simulink library "mfcm_block_lib_v1"  (Simulink 6.1)
undefined symbols (not defined in the file or in its folder): calc_path_data, mfcm_add_phase_noise, mfcm_delay_line_depth, mfcm_dpram_format_init, mfcm_dpram_format_lsb, mfcm_dpram_format_width, mfcm_matrix_rom, mfcm_phase_noise_pacc, mfcm_phase_noise_pinc, mfcm_spectrum_roms
libraries: xbsIndex_r4 x234, mfcm_misc_lib_v1 x8, mfcm_block_lib_v1 x4, mfcm_vector_lib_v1 x3, xbsCopyrightNotice_r4 x1
(part 1 of 3)
settings Model: Creator=dandrews  LastModifiedBy=alexc

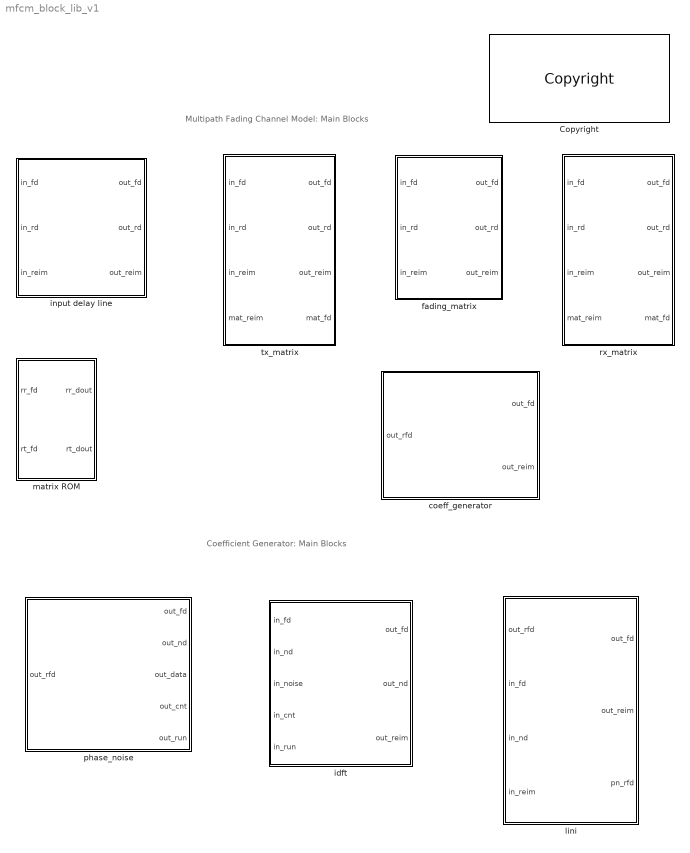
== system mfcm_block_lib_v1 ==
  note: Multipath Fading Channel Model: Main Blocks
  note: Coefficient Generator: Main Blocks
  Copyright : xbsCopyrightNotice_r4/Copyright
  coeff_generator : Subsystem  mask{RATE=32, OUT_WIDTH=18, OUT_BINPT=15, TRIG_WIDTH=18, SPEC_DATA=calc_path_data([2 2 2 2],[1 1 1 1]), SPEC_WIDTH=17, SPEC_BINPT=16, SEED='461AF8228C9F8C92', N_OSC=64, N_IDFT=8192}
      mask prompts: OUT_WIDTH "Output Width"; OUT_BINPT "Output Binary Point"; TRIG_WIDTH "Twiddle Factor Width"; SPEC_DATA "Spectrum Data"; SPEC_WIDTH "Spectrum Width"; SPEC_BINPT "Spectrum Binary Point"; SEED "Random Seed"
      mask Display:
      | disp(sprintf('z^{-14}\nPATHS=%d',prod(size(SPEC_DATA))),'texmode','on');
      | 
      | port_label('input',1,'out_rfd');
      | 
      | port_label('output',1,'out_fd');
      | port_label('output',2,'out_reim');
  fading_matrix : Subsystem  mask{RATE=64, DATAPATH_WIDTH=18, OUT_BINPT=15, SPEC_DATA=calc_path_data([1],[1]), SEED='461AF8228C9F8C92'}
      mask prompts: DATAPATH_WIDTH "Datapath Width"; OUT_BINPT "Output Binary Point"; SPEC_DATA "Spectrum Data"; SEED "Random Seed"
  idft : Subsystem  mask{OUT_WIDTH=18, OUT_BINPT=15, TRIG_WIDTH=18, SPEC_DATA=calc_path_data([3 2 1 0],[1 1 1 1]), SPEC_WIDTH=17, SPEC_BINPT=16, N_OSC=64, N_IDFT=8192}
      mask prompts: OUT_WIDTH "Output Width"; OUT_BINPT "Output Binary Point"; TRIG_WIDTH "Twiddle Factor Width"; SPEC_DATA "Spectrum Data"; SPEC_WIDTH "Spectrum Width"; SPEC_BINPT "Spectrum Binary Point"
  input delay line : Subsystem  mask{MT=4, DELAY=[0 1 2]}
      mask prompts: MT "Number of Transmit Antennas"; DELAY "Path Delay Vector"
  lini : Subsystem  mask{RATE=64, OUT_WIDTH=18, OUT_BINPT=15, CHANNELS=16}
      mask prompts: OUT_WIDTH "Output Width"; OUT_BINPT "Output Binary Point"; CHANNELS "Number Of Channels"
  matrix ROM : Subsystem  mask{MATS=mfcm_matrix_rom(eye(4),1,eye(4)), DATAPATH_WIDTH=18, MAT_BINPT=17}
      mask prompts: MATS "Matrix ROM Data"; DATAPATH_WIDTH "Datapath Width in Bits"; MAT_BINPT "Transmit/Receive Matrix Binary Point"
      mask Display:
      | disp('z^{-3}','texmode','on');
      | 
      | port_label('input',1,'rr_fd');
      | port_label('input',2,'rt_fd');
      | port_label('output',1,'rr_dout');
      | port_label('output',2,'rt_dout');
  phase_noise : Subsystem  mask{SPEC_DATA=calc_path_data([3 2 1 0],[1 1 1 1]), SEED='461AF8228C9F8C92', N_OSC=64, N_IDFT=8192}
      mask prompts: SPEC_DATA "Spectrum Data (with phase noise)"; SEED "Random Seed"
  rx_matrix : Subsystem  mask{MR=4, N=3, BYPASS=0, WIDTH=18, BINPT=15}
      mask prompts: MR "Number of Rx Antennas"; N "Number of Paths"; WIDTH "Output Width"; BINPT "Output Binary Point"
  tx_matrix : Subsystem  mask{MT=4, N=3, BYPASS=0, WIDTH=18, BINPT=17}
      mask prompts: MT "Number of Tx Antennas"; N "Number of Paths"; WIDTH "Output Width"; BINPT "Output Binary Point"

== system mfcm_block_lib_v1/coeff_generator ==
  out_rfd : Inport  Port=1  LatchInput=off
  " Copyright" : Subsystem  mask(Xilinx Digital Up Converter Copyright){}
      mask init:
      | iPos = get_param(gcb,'Position');
      | iWidth=iPos(3)-iPos(1); iHeight=iPos(4)-iPos(2);
      | iCx=iWidth/2;
      | iCy=iHeight/2;
      | [logoX, logoY] = xlogo(iPos);
      mask Display: patch(logoX,logoY, [0.56 0.36 0.27]);
  idft : mfcm_block_lib_v1/idft  OUT_WIDTH=OUT_WIDTH  OUT_BINPT=OUT_BINPT  TRIG_WIDTH=TRIG_WIDTH  SPEC_DATA=SPEC_DATA  SPEC_WIDTH=SPEC_WIDTH  SPEC_BINPT=SPEC_BINPT  N_OSC=N_OSC  N_IDFT=N_IDFT
  lini : mfcm_block_lib_v1/lini  RATE=RATE  OUT_WIDTH=OUT_WIDTH  OUT_BINPT=OUT_BINPT  CHANNELS=prod(size(SPEC_DATA))
  phase_noise : mfcm_block_lib_v1/phase_noise  SPEC_DATA=mfcm_add_phase_noise(SPEC_DATA,SEED)  SEED=SEED  N_OSC=N_OSC  N_IDFT=N_IDFT
  out_fd : Outport
  out_reim : Outport  Port=2
  wires:
  phase_noise/3 -> idft/3
  lini/3 -> phase_noise/1
  out_rfd/1 -> lini/1
  lini/2 -> out_reim/1
  lini/1 -> out_fd/1
  idft/3 -> lini/4
  idft/2 -> lini/3
  idft/1 -> lini/2
  phase_noise/2 -> idft/2
  phase_noise/4 -> idft/4
  phase_noise/1 -> idft/1
  phase_noise/5 -> idft/5

== system mfcm_block_lib_v1/fading_matrix ==
  in_fd : Inport  Port=1  LatchInput=off
  in_rd : Inport  Port=2  LatchInput=off
  in_reim : Inport  Port=3  LatchInput=off
  Terminator : Terminator
  cg : mfcm_block_lib_v1/coeff_generator  RATE=RATE  OUT_WIDTH=DATAPATH_WIDTH  OUT_BINPT=OUT_BINPT  TRIG_WIDTH=DATAPATH_WIDTH  SPEC_DATA=permute(SPEC_DATA,[2 1 3])  SPEC_WIDTH=DATAPATH_WIDTH-1  SPEC_BINPT=DATAPATH_WIDTH-2  SEED=SEED  N_OSC=64  N_IDFT=8192
  fd_pipe : xbsIndex_r4/Delay  en=off  latency=14  dbl_ovrd=off  reg_retiming=off  block_type=delay
      settings: infoedit="Delay line having  configurable length.<P><P>Hardware notes: A delay line is a chain, each link of which is an SRL16 followed by a flip-flop. If register retiming is enabled, the delay line is a chain of flip-flops."  xl_area=[0, 0, 0, 0, 0, 0, 0]  block_version=VER_STRING_GOES_HERE
  multiply SCMAT by SCVEC : mfcm_vector_lib_v1/multiply SCMAT by SCVEC  MAT_H=size(SPEC_DATA,1)*size(SPEC_DATA,3)  MAT_W=size(SPEC_DATA,2)  OUT_WIDTH=DATAPATH_WIDTH  OUT_BINPT=OUT_BINPT
  rd_pipe : xbsIndex_r4/Delay  en=off  latency=14  dbl_ovrd=off  reg_retiming=off  block_type=delay
      settings: infoedit="Delay line having  configurable length.<P><P>Hardware notes: A delay line is a chain, each link of which is an SRL16 followed by a flip-flop. If register retiming is enabled, the delay line is a chain of flip-flops."  xl_area=[0, 0, 0, 0, 0, 0, 0]  block_version=VER_STRING_GOES_HERE
  reim_pipe : xbsIndex_r4/Delay  en=off  latency=14  dbl_ovrd=off  reg_retiming=off  block_type=delay
      settings: infoedit="Delay line having  configurable length.<P><P>Hardware notes: A delay line is a chain, each link of which is an SRL16 followed by a flip-flop. If register retiming is enabled, the delay line is a chain of flip-flops."  xl_area=[0, 0, 0, 0, 0, 0, 0]  block_version=VER_STRING_GOES_HERE
  out_fd : Outport
  out_rd : Outport  Port=2
  out_reim : Outport  Port=3
  wires:
  in_fd/1 -> fd_pipe/1, cg/1
  in_reim/1 -> reim_pipe/1
  in_rd/1 -> rd_pipe/1
  fd_pipe/1 -> multiply SCMAT by SCVEC/1
  rd_pipe/1 -> multiply SCMAT by SCVEC/2
  reim_pipe/1 -> multiply SCMAT by SCVEC/3
  multiply SCMAT by SCVEC/1 -> out_fd/1
  multiply SCMAT by SCVEC/2 -> out_rd/1
  multiply SCMAT by SCVEC/3 -> out_reim/1
  cg/1 -> Terminator/1
  cg/2 -> multiply SCMAT by SCVEC/4

== system mfcm_block_lib_v1/idft ==
  note: iDFT engine has lataency of 8
  in_fd : Inport  Port=1  LatchInput=off
  in_nd : Inport  Port=2  LatchInput=off
  in_noise : Inport  Port=3  LatchInput=off
  in_cnt : Inport  Port=4  LatchInput=off
  in_run : Inport  Port=5  LatchInput=off
  fd_pipe : xbsIndex_r4/Delay  en=off  latency=8+4+2  dbl_ovrd=off  reg_retiming=off  block_type=delay
      settings: infoedit="Delay line having  configurable length.<P><P>Hardware notes: A delay line is a chain, each link of which is an SRL16 followed by a flip-flop. If register retiming is enabled, the delay line is a chain of flip-flops."  xl_area=[0, 0, 0, 0, 0, 0, 0]  block_version=VER_STRING_GOES_HERE
  idft_control : Subsystem
  idft_engine : Subsystem
  nd_pipe : xbsIndex_r4/Delay  en=off  latency=8+4+2  dbl_ovrd=off  reg_retiming=off  block_type=delay
      settings: infoedit="Delay line having  configurable length.<P><P>Hardware notes: A delay line is a chain, each link of which is an SRL16 followed by a flip-flop. If register retiming is enabled, the delay line is a chain of flip-flops."  xl_area=[0, 0, 0, 0, 0, 0, 0]  block_version=VER_STRING_GOES_HERE
  out_pipe : xbsIndex_r4/Delay  en=off  latency=1  dbl_ovrd=off  reg_retiming=off  block_type=delay
      settings: infoedit="Delay line having  configurable length.<P><P>Hardware notes: A delay line is a chain, each link of which is an SRL16 followed by a flip-flop. If register retiming is enabled, the delay line is a chain of flip-flops."  xl_area=[0, 0, 0, 0, 0, 0, 0]  block_version=VER_STRING_GOES_HERE
  safe_mac : mfcm_misc_lib_v1/safe_mac  ACC_GROWTH=log2(N_OSC)  ACC_DEPTH=2
  sat_convert : xbsIndex_r4/Convert  arith_type="Signed  (2's comp)"  n_bits=OUT_WIDTH  bin_pt=OUT_BINPT  quantization=Truncate  overflow=Saturate  latency=1  dbl_ovrd=off  pipeline=off  block_type=convert
      settings: infoedit=The input is presented at the output after quantization and overflow effects.<P><P>Hardware notes: Additional hardware is used when rounding or saturation is selected and output width is less than the input width.  block_version=VER_STRING_GOES_HERE
  out_fd : Outport
  out_nd : Outport  Port=2
  out_reim : Outport  Port=3
  wires:
  idft_engine/4(mac_sub) -> safe_mac/4
  idft_engine/3(mac_acc) -> safe_mac/3
  idft_engine/2(mac_trig) -> safe_mac/2
  idft_engine/1(mac_gain) -> safe_mac/1
  idft_control/3(sin_not_cos) -> idft_engine/3(sin_not_cos)
  idft_control/5(out_kne0) -> idft_engine/5(in_kne0)
  fd_pipe/1 -> out_fd/1
  idft_control/7(out_fd) -> fd_pipe/1
  nd_pipe/1 -> out_nd/1
  idft_control/8(out_kmax) -> nd_pipe/1
  sat_convert/1 -> out_reim/1
  safe_mac/1 -> out_pipe/1
  idft_control/6(out_n) -> idft_engine/6(in_n)
  in_cnt/1 -> idft_control/4(in_cnt)
  in_noise/1 -> idft_control/3(in_noise)
  in_nd/1 -> idft_control/2(in_nd)
  in_fd/1 -> idft_control/1(in_fd)
  idft_control/1(spec_freq) -> idft_engine/1(spec_freq)
  idft_control/4(spec_noise) -> idft_engine/4(spec_noise)
  idft_control/2(spec_path) -> idft_engine/2(spec_path)
  in_run/1 -> idft_control/5(run)
  out_pipe/1 -> sat_convert/1

== system mfcm_block_lib_v1/input delay line ==
  in_fd : Inport  Port=1  LatchInput=off
  in_rd : Inport  Port=2  LatchInput=off
  in_reim : Inport  Port=3  LatchInput=off
  dpram : mfcm_misc_lib_v1/dpram  MEM_DEPTH=mfcm_delay_line_depth(DELAY,MT)  MEM_INIT=0  MEM_MAXDEPTH=16
  pipe0 : xbsIndex_r4/Delay  en=off  latency=2  dbl_ovrd=off  reg_retiming=off  block_type=delay
      settings: infoedit="Delay line having  configurable length.<P><P>Hardware notes: A delay line is a chain, each link of which is an SRL16 followed by a flip-flop. If register retiming is enabled, the delay line is a chain of flip-flops."  xl_area=[0, 0, 0, 0, 0, 0, 0]  block_version=VER_STRING_GOES_HERE
  pipe1 : xbsIndex_r4/Delay  en=on  latency=2  dbl_ovrd=off  reg_retiming=off  block_type=delay
      settings: infoedit="Delay line having  configurable length.<P><P>Hardware notes: A delay line is a chain, each link of which is an SRL16 followed by a flip-flop. If register retiming is enabled, the delay line is a chain of flip-flops."  xl_area=[0, 0, 0, 0, 0, 0, 0]  block_version=VER_STRING_GOES_HERE
  read_control : Subsystem
  write_control : Subsystem
  out_fd : Outport
  out_rd : Outport  Port=2
  out_reim : Outport  Port=3
  wires:
  read_control/3(rd_en) -> pipe1/2
  read_control/2(rd_rd) -> pipe1/1
  pipe1/1 -> out_rd/1
  write_control/1(rd_fd) -> read_control/1(in_fd)
  pipe0/1 -> out_fd/1
  read_control/1(rd_fd) -> pipe0/1
  read_control/4(rd_add) -> dpram/1
  dpram/1 -> out_reim/1
  write_control/4(wr_en) -> dpram/4
  write_control/3(wr_data) -> dpram/3
  write_control/2(wr_add) -> dpram/2
  in_rd/1 -> write_control/2(in_rd)
  in_fd/1 -> write_control/1(in_fd)
  in_reim/1 -> write_control/3(in_reim)

== system mfcm_block_lib_v1/lini ==
  out_rfd : Inport  Port=1  LatchInput=off
  in_fd : Inport  Port=2  LatchInput=off
  in_nd : Inport  Port=3  LatchInput=off
  in_reim : Inport  Port=4  LatchInput=off
  lini_engine : Subsystem
  lini_fifo : Subsystem
  rate_counter : Subsystem
  out_fd : Outport
  out_reim : Outport  Port=2
  pn_rfd : Outport  Port=3
  wires:
  in_fd/1 -> lini_fifo/1(in_fd)
  in_nd/1 -> lini_fifo/2(in_nd)
  in_reim/1 -> lini_fifo/3(in_reim)
  lini_fifo/2(out_re) -> lini_engine/2(in_re)
  lini_fifo/3(out_im) -> lini_engine/3(in_im)
  lini_fifo/5(out_b) -> lini_engine/5(in_b)
  lini_fifo/1(lini_fd) -> lini_engine/1(in_fd)
  lini_engine/1(out_fd) -> out_fd/1
  lini_engine/2(out_reim) -> out_reim/1
  out_rfd/1 -> rate_counter/1(en)
  rate_counter/1(lini_rfd) -> lini_fifo/4(lini_rfd)
  rate_counter/2(pn_rfd) -> lini_fifo/5(pn_rfd), pn_rfd/1
  lini_fifo/6(pn_fd) -> lini_engine/6(pn_fd)
  lini_fifo/4(valid) -> lini_engine/4(in_valid)

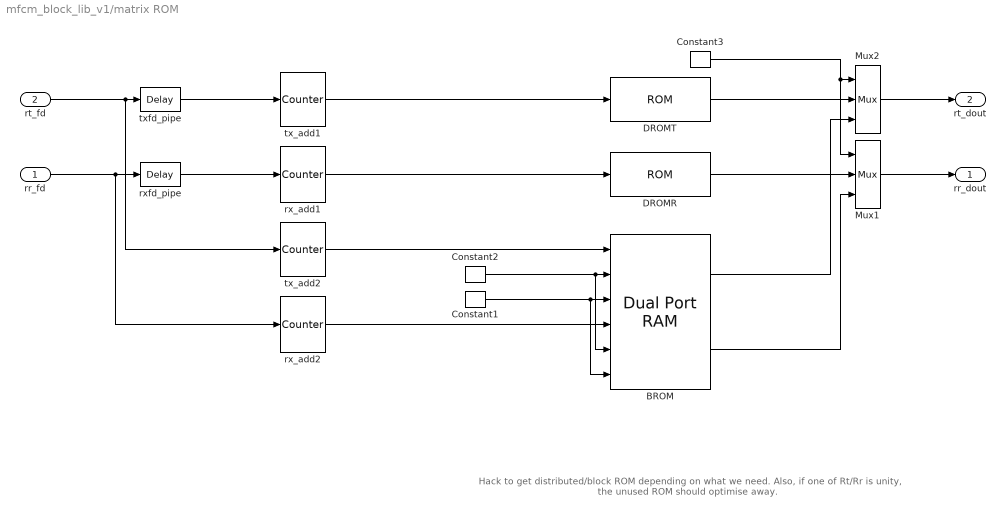
== system mfcm_block_lib_v1/matrix ROM ==
  note: Hack to get distributed/block ROM depending on what we need.
      | Also, if one of Rt/Rr is unity, the unused ROM should optimise away.
  rr_fd : Inport  Port=1  LatchInput=off
  rt_fd : Inport  Port=2  LatchInput=off
  BROM : xbsIndex_r4/Dual Port RAM  depth=2^ceil(log2(max(length(MATS.brom),2)))  initVector=MATS.brom  distributed_mem=Block RAM  init_a=0  init_b=0  rst_a=off  rst_b=off  en_a=off  en_b=off  latency=2  write_mode_A=Read After Write  write_mode_B=Read After Write  dbl_ovrd=off  use_rpm=on  block_type=dpram
      settings: block_version=VER_STRING_GOES_HERE
  Constant1 : xbsIndex_r4/Constant  arith_type=Boolean  const=0  n_bits=1  bin_pt=0  explicit_period=off  period=1  equ=P=C  opselect=C  inp2=PCIN>>17  opr=+  inp1=P  carry=CIN  dbl_ovrd=off  block_type=constant
      settings: block_version=VER_STRING_GOES_HERE
  Constant2 : xbsIndex_r4/Constant  arith_type=Signed (2's comp)  const=0  n_bits=DATAPATH_WIDTH  bin_pt=MAT_BINPT  explicit_period=off  period=1  equ=P=C  opselect=C  inp2=PCIN>>17  opr=+  inp1=P  carry=CIN  dbl_ovrd=off  block_type=constant
      settings: block_version=VER_STRING_GOES_HERE
  Constant3 : xbsIndex_r4/Constant  arith_type=Boolean  const=double(MATS.use_bram~=0)  n_bits=1  bin_pt=0  explicit_period=off  period=1  equ=P=C  opselect=C  inp2=PCIN>>17  opr=+  inp1=P  carry=CIN  dbl_ovrd=off  block_type=constant
      settings: block_version=VER_STRING_GOES_HERE
  DROMR : xbsIndex_r4/ROM  depth=2^ceil(log2(max(length(MATS.dromr),2)))  initVector=MATS.dromr  distributed_mem=Distributed memory  rst=off  init_reg=0  en=off  latency=1  arith_type="Signed  (2's comp)"  n_bits=DATAPATH_WIDTH  bin_pt=MAT_BINPT  dbl_ovrd=off  use_rpm=on  block_type=sprom
      settings: xl_area=[0, 0, 0, 0, 0, 0, 0]  block_version=VER_STRING_GOES_HERE
  DROMT : xbsIndex_r4/ROM  depth=2^ceil(log2(max(length(MATS.dromt),2)))  initVector=MATS.dromt  distributed_mem=Distributed memory  rst=off  init_reg=0  en=off  latency=1  arith_type="Signed  (2's comp)"  n_bits=DATAPATH_WIDTH  bin_pt=MAT_BINPT  dbl_ovrd=off  use_rpm=on  block_type=sprom
      settings: xl_area=[0, 0, 0, 0, 0, 0, 0]  block_version=VER_STRING_GOES_HERE
  Mux1 : xbsIndex_r4/Mux  inputs=2  en=off  latency=0  precision=Full  arith_type=Unsigned  n_bits=8  bin_pt=2  quantization=Truncate  overflow=Wrap  dbl_ovrd=off  block_type=mux
      settings: block_version=VER_STRING_GOES_HERE
  Mux2 : xbsIndex_r4/Mux  inputs=2  en=off  latency=0  precision=Full  arith_type=Unsigned  n_bits=8  bin_pt=2  quantization=Truncate  overflow=Wrap  dbl_ovrd=off  block_type=mux
      settings: block_version=VER_STRING_GOES_HERE
  rx_add1 : xbsIndex_r4/Counter  cnt_type=Free Running  cnt_to=0  operation=Up  start_count=0  cnt_by_val=1  arith_type=Unsigned  n_bits=ceil(log2(max(length(MATS.dromr),2)))  bin_pt=0  load_pin=off  rst=on  en=off  dbl_ovrd=off  explicit_period=off  period=2  block_type=counter
      settings: infoedit="Configurable up, down and up/down counter.<P><P>Hardware notes: Free running counters are the least expensive in hardware.  A count limited counter is implemented by combining a counter with a comparator."  xl_area=[0, 0, 0, 0, 0, 0, 0]  block_version=VER_STRING_GOES_HERE
  rx_add2 : xbsIndex_r4/Counter  cnt_type=Free Running  cnt_to=0  operation=Up  start_count=MATS.brom_rr  cnt_by_val=1  arith_type=Unsigned  n_bits=ceil(log2(max(length(MATS.brom),2)))  bin_pt=0  load_pin=off  rst=on  en=off  dbl_ovrd=off  explicit_period=off  period=2  block_type=counter
      settings: infoedit="Configurable up, down and up/down counter.<P><P>Hardware notes: Free running counters are the least expensive in hardware.  A count limited counter is implemented by combining a counter with a comparator."  xl_area=[0, 0, 0, 0, 0, 0, 0]  block_version=VER_STRING_GOES_HERE
  rxfd_pipe : xbsIndex_r4/Delay  en=off  latency=1  dbl_ovrd=off  reg_retiming=off  block_type=delay
      settings: infoedit="Delay line having  configurable length.<P><P>Hardware notes: A delay line is a chain, each link of which is an SRL16 followed by a flip-flop. If register retiming is enabled, the delay line is a chain of flip-flops."  block_version=VER_STRING_GOES_HERE
  tx_add1 : xbsIndex_r4/Counter  cnt_type=Free Running  cnt_to=Inf  operation=Up  start_count=0  cnt_by_val=1  arith_type=Unsigned  n_bits=ceil(log2(max(length(MATS.dromt),2)))  bin_pt=0  load_pin=off  rst=on  en=off  dbl_ovrd=off  explicit_period=off  period=2  block_type=counter
      settings: infoedit="Configurable up, down and up/down counter.<P><P>Hardware notes: Free running counters are the least expensive in hardware.  A count limited counter is implemented by combining a counter with a comparator."  xl_area=[0, 0, 0, 0, 0, 0, 0]  block_version=VER_STRING_GOES_HERE
  tx_add2 : xbsIndex_r4/Counter  cnt_type=Free Running  cnt_to=Inf  operation=Up  start_count=MATS.brom_rt  cnt_by_val=1  arith_type=Unsigned  n_bits=ceil(log2(max(length(MATS.brom),2)))  bin_pt=0  load_pin=off  rst=on  en=off  dbl_ovrd=off  explicit_period=off  period=2  block_type=counter
      settings: infoedit="Configurable up, down and up/down counter.<P><P>Hardware notes: Free running counters are the least expensive in hardware.  A count limited counter is implemented by combining a counter with a comparator."  xl_area=[0, 0, 0, 0, 0, 0, 0]  block_version=VER_STRING_GOES_HERE
  txfd_pipe : xbsIndex_r4/Delay  en=off  latency=1  dbl_ovrd=off  reg_retiming=off  block_type=delay
      settings: infoedit="Delay line having  configurable length.<P><P>Hardware notes: A delay line is a chain, each link of which is an SRL16 followed by a flip-flop. If register retiming is enabled, the delay line is a chain of flip-flops."  block_version=VER_STRING_GOES_HERE
  rr_dout : Outport
  rt_dout : Outport  Port=2
  wires:
  Constant1/1 -> BROM/6, BROM/3
  Constant2/1 -> BROM/5, BROM/2
  DROMR/1 -> Mux1/2
  DROMT/1 -> Mux2/2
  rr_fd/1 -> rx_add2/1, rxfd_pipe/1
  rt_fd/1 -> tx_add2/1, txfd_pipe/1
  rxfd_pipe/1 -> rx_add1/1
  tx_add1/1 -> DROMT/1
  txfd_pipe/1 -> tx_add1/1
  BROM/1 -> Mux2/3
  BROM/2 -> Mux1/3
  Mux2/1 -> rt_dout/1
  Mux1/1 -> rr_dout/1
  rx_add1/1 -> DROMR/1
  Constant3/1 -> Mux2/1, Mux1/1
  tx_add2/1 -> BROM/1
  rx_add2/1 -> BROM/4

== system mfcm_block_lib_v1/phase_noise ==
  note: lfsr must be clocked once per path.
      | Note that this does not need to be synchronised to pn_engine block
      | - if they are not synced there is a very small chance that two increments
      | can be updated per path - this is harmless and on average will be fine.
  out_rfd : Inport  Port=1  LatchInput=off
  Constant1 : xbsIndex_r4/Constant  arith_type=Unsigned  const=1  n_bits=1  bin_pt=0  explicit_period=off  period=1  equ=P=C  opselect=C  inp2=PCIN>>17  opr=+  inp1=P  carry=CIN  dbl_ovrd=off  block_type=constant
      settings: block_version=VER_STRING_GOES_HERE
  Slice : xbsIndex_r4/Slice  nbits=ceil(log2(2*N_OSC))  boolean_output=off  mode=Lower Bit Location + Width  bit1=0  base1=MSB of Input  bit0=0  base0=LSB of Input  dbl_ovrd=off  block_type=slice
      settings: infoedit="Extracts a given range of bits from each input sample and presents it at the output.  The output type is ordinarily unsigned with binary point at zero, but can be Boolean when the slice is one bit wide.<P><P>Hardware notes: In hardware this block costs nothing."  block_version=VER_STRING_GOES_HERE
  lfsr1 : Subsystem  mask{SEED=SEED}
      mask prompts: SEED "Seed value (16 hex digits)"
  lfsr_relop : xbsIndex_r4/Relational  mode=a=b  en=off  latency=1  dbl_ovrd=off  block_type=relational
      settings: xl_area=[0, 0, 0, 0, 0, 0, 0]  block_version=VER_STRING_GOES_HERE
  pn_engine : Subsystem
  out_fd : Outport
  out_nd : Outport  Port=2
  out_data : Outport  Port=3
  out_cnt : Outport  Port=4
  out_run : Outport  Port=5
  wires:
  pn_engine/5(out_run) -> out_run/1
  pn_engine/1(out_fd) -> out_fd/1
  pn_engine/3(out_data) -> out_data/1
  lfsr1/1(out_data) -> pn_engine/2(noise)
  out_rfd/1 -> pn_engine/1(rfd)
  pn_engine/2(out_nd) -> out_nd/1
  pn_engine/4(out_cnt) -> out_cnt/1, Slice/1
  lfsr_relop/1 -> lfsr1/1(en)
  Constant1/1 -> lfsr_relop/2
  Slice/1 -> lfsr_relop/1

== system mfcm_block_lib_v1/rx_matrix ==
  note: Matrix ROM
      | latency is 3
  note: Bypass path - if RR is unity we don't need all this.
      | Should optimise away
  in_fd : Inport  Port=1  LatchInput=off
  in_rd : Inport  Port=2  LatchInput=off
  in_reim : Inport  Port=3  LatchInput=off
  mat_reim : Inport  Port=4  LatchInput=off
  Constant1 : xbsIndex_r4/Constant  arith_type=Boolean  const=double(BYPASS~=0)  n_bits=1  bin_pt=0  explicit_period=off  period=1  equ=P=C  opselect=C  inp2=PCIN>>17  opr=+  inp1=P  carry=CIN  dbl_ovrd=off  block_type=constant
      settings: block_version=VER_STRING_GOES_HERE
  Convert : xbsIndex_r4/Convert  arith_type="Signed  (2's comp)"  n_bits=WIDTH  bin_pt=BINPT  quantization=Truncate  overflow=Wrap  latency=0  dbl_ovrd=off  pipeline=off  block_type=convert
      settings: infoedit=The input is presented at the output after quantization and overflow effects.<P><P>Hardware notes: Additional hardware is used when rounding or saturation is selected and output width is less than the input width.  xl_area=[0, 0, 0, 0, 0, 0, 0]  block_version=VER_STRING_GOES_HERE
  Mux1 : xbsIndex_r4/Mux  inputs=2  en=off  latency=0  precision=Full  arith_type=Unsigned  n_bits=8  bin_pt=2  quantization=Truncate  overflow=Wrap  dbl_ovrd=off  block_type=mux
      settings: block_version=VER_STRING_GOES_HERE
  Mux2 : xbsIndex_r4/Mux  inputs=2  en=off  latency=0  precision=Full  arith_type=Unsigned  n_bits=8  bin_pt=2  quantization=Truncate  overflow=Wrap  dbl_ovrd=off  block_type=mux
      settings: block_version=VER_STRING_GOES_HERE
  Mux3 : xbsIndex_r4/Mux  inputs=2  en=off  latency=0  precision=Full  arith_type=Unsigned  n_bits=8  bin_pt=2  quantization=Truncate  overflow=Wrap  dbl_ovrd=off  block_type=mux
      settings: block_version=VER_STRING_GOES_HERE
  fd_pipe : xbsIndex_r4/Delay  en=off  latency=3  dbl_ovrd=off  reg_retiming=off  block_type=delay
      settings: infoedit="Delay line having  configurable length.<P><P>Hardware notes: A delay line is a chain, each link of which is an SRL16 followed by a flip-flop. If register retiming is enabled, the delay line is a chain of flip-flops."  xl_area=[0, 0, 0, 0, 0, 0, 0]  block_version=VER_STRING_GOES_HERE
  multiply SCMAT by SCVEC : mfcm_vector_lib_v1/multiply SCMAT by SCVEC  MAT_H=MR  MAT_W=MR*N  OUT_WIDTH=WIDTH  OUT_BINPT=BINPT
  rd_pipe : xbsIndex_r4/Delay  en=off  latency=3  dbl_ovrd=off  reg_retiming=off  block_type=delay
      settings: infoedit="Delay line having  configurable length.<P><P>Hardware notes: A delay line is a chain, each link of which is an SRL16 followed by a flip-flop. If register retiming is enabled, the delay line is a chain of flip-flops."  xl_area=[0, 0, 0, 0, 0, 0, 0]  block_version=VER_STRING_GOES_HERE
  reim_pipe : xbsIndex_r4/Delay  en=off  latency=3  dbl_ovrd=off  reg_retiming=off  block_type=delay
      settings: infoedit="Delay line having  configurable length.<P><P>Hardware notes: A delay line is a chain, each link of which is an SRL16 followed by a flip-flop. If register retiming is enabled, the delay line is a chain of flip-flops."  xl_area=[0, 0, 0, 0, 0, 0, 0]  block_version=VER_STRING_GOES_HERE
  out_fd : Outport
  out_rd : Outport  Port=2
  out_reim : Outport  Port=3
  mat_fd : Outport  Port=4
  wires:
  reim_pipe/1 -> multiply SCMAT by SCVEC/3
  rd_pipe/1 -> multiply SCMAT by SCVEC/2
  in_rd/1 -> rd_pipe/1, Mux1/3
  mat_reim/1 -> multiply SCMAT by SCVEC/4
  in_fd/1 -> fd_pipe/1, Mux2/3, mat_fd/1
  in_reim/1 -> reim_pipe/1, Convert/1
  fd_pipe/1 -> multiply SCMAT by SCVEC/1
  multiply SCMAT by SCVEC/1 -> Mux2/2
  multiply SCMAT by SCVEC/2 -> Mux1/2
  multiply SCMAT by SCVEC/3 -> Mux3/2
  Constant1/1 -> Mux1/1, Mux3/1, Mux2/1
  Mux2/1 -> out_fd/1
  Mux1/1 -> out_rd/1
  Mux3/1 -> out_reim/1
  Convert/1 -> Mux3/3

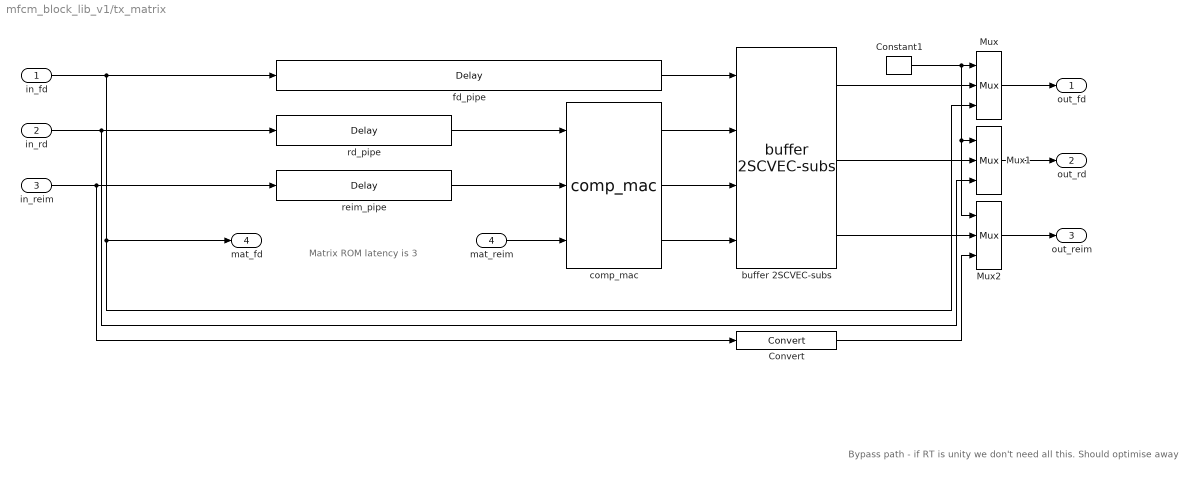
== system mfcm_block_lib_v1/tx_matrix ==
  note: Matrix ROM
      | latency is 3
  note: Bypass path - if RT is unity we don't need all this.
      | Should optimise away
  in_fd : Inport  Port=1  LatchInput=off
  in_rd : Inport  Port=2  LatchInput=off
  in_reim : Inport  Port=3  LatchInput=off
  mat_reim : Inport  Port=4  LatchInput=off
  Constant1 : xbsIndex_r4/Constant  arith_type=Boolean  const=double(BYPASS~=0)  n_bits=1  bin_pt=0  explicit_period=off  period=1  equ=P=C  opselect=C  inp2=PCIN>>17  opr=+  inp1=P  carry=CIN  dbl_ovrd=off  block_type=constant
      settings: block_version=VER_STRING_GOES_HERE
  Convert : xbsIndex_r4/Convert  arith_type="Signed  (2's comp)"  n_bits=WIDTH  bin_pt=BINPT  quantization=Truncate  overflow=Wrap  latency=0  dbl_ovrd=off  pipeline=off  block_type=convert
      settings: infoedit=The input is presented at the output after quantization and overflow effects.<P><P>Hardware notes: Additional hardware is used when rounding or saturation is selected and output width is less than the input width.  xl_area=[0, 0, 0, 0, 0, 0, 0]  block_version=VER_STRING_GOES_HERE
  Mux : xbsIndex_r4/Mux  inputs=2  en=off  latency=0  precision=Full  arith_type=Unsigned  n_bits=8  bin_pt=2  quantization=Truncate  overflow=Wrap  dbl_ovrd=off  block_type=mux
      settings: block_version=VER_STRING_GOES_HERE
  Mux1 : xbsIndex_r4/Mux  inputs=2  en=off  latency=0  precision=Full  arith_type=Unsigned  n_bits=8  bin_pt=2  quantization=Truncate  overflow=Wrap  dbl_ovrd=off  block_type=mux
      settings: block_version=VER_STRING_GOES_HERE
  Mux2 : xbsIndex_r4/Mux  inputs=2  en=off  latency=0  precision=Full  arith_type=Unsigned  n_bits=8  bin_pt=2  quantization=Truncate  overflow=Wrap  dbl_ovrd=off  block_type=mux
      settings: block_version=VER_STRING_GOES_HERE
  buffer 2SCVEC-subs : mfcm_vector_lib_v1/buffer 2SCVEC-subs  SUB_SIZE=MT  SUB_COUNT=N  REP_COUNT=MT
  comp_mac : mfcm_misc_lib_v1/comp_mac  MULS=MT  OUT_WIDTH=WIDTH  OUT_BINPT=BINPT
  fd_pipe : xbsIndex_r4/Delay  en=off  latency=3+2*MT+8  dbl_ovrd=off  reg_retiming=off  block_type=delay
      settings: infoedit="Delay line having  configurable length.<P><P>Hardware notes: A delay line is a chain, each link of which is an SRL16 followed by a flip-flop. If register retiming is enabled, the delay line is a chain of flip-flops."  xl_area=[0, 0, 0, 0, 0, 0, 0]  block_version=VER_STRING_GOES_HERE
  rd_pipe : xbsIndex_r4/Delay  en=off  latency=3  dbl_ovrd=off  reg_retiming=off  block_type=delay
      settings: infoedit="Delay line having  configurable length.<P><P>Hardware notes: A delay line is a chain, each link of which is an SRL16 followed by a flip-flop. If register retiming is enabled, the delay line is a chain of flip-flops."  xl_area=[0, 0, 0, 0, 0, 0, 0]  block_version=VER_STRING_GOES_HERE
  reim_pipe : xbsIndex_r4/Delay  en=off  latency=3  dbl_ovrd=off  reg_retiming=off  block_type=delay
      settings: infoedit="Delay line having  configurable length.<P><P>Hardware notes: A delay line is a chain, each link of which is an SRL16 followed by a flip-flop. If register retiming is enabled, the delay line is a chain of flip-flops."  xl_area=[0, 0, 0, 0, 0, 0, 0]  block_version=VER_STRING_GOES_HERE
  out_fd : Outport
  out_rd : Outport  Port=2
  out_reim : Outport  Port=3
  mat_fd : Outport  Port=4
  wires:
  in_reim/1 -> reim_pipe/1, Convert/1
  buffer 2SCVEC-subs/1 -> Mux/2
  buffer 2SCVEC-subs/2 -> Mux1/2
  buffer 2SCVEC-subs/3 -> Mux2/2
  in_fd/1 -> fd_pipe/1, Mux/3, mat_fd/1
  mat_reim/1 -> comp_mac/3
  in_rd/1 -> rd_pipe/1, Mux1/3
  rd_pipe/1 -> comp_mac/1
  reim_pipe/1 -> comp_mac/2
  fd_pipe/1 -> buffer 2SCVEC-subs/1
  comp_mac/1 -> buffer 2SCVEC-subs/2
  comp_mac/2 -> buffer 2SCVEC-subs/3
  comp_mac/3 -> buffer 2SCVEC-subs/4
  Constant1/1 -> Mux1/1, Mux2/1, Mux/1
  Mux/1 -> out_fd/1
  Mux1/1 -> out_rd/1
  Mux2/1 -> out_reim/1
  Convert/1 -> Mux2/3

== system mfcm_block_lib_v1/coeff_generator/ Copyright ==
  note: -- Copyright(C) 2005 by Xilinx, Inc. All rights reserved.
      |  -- This text/file contains proprietary, confidential
      |  -- information of Xilinx, Inc., is distributed under license
      |  -- from Xilinx, Inc., and may be used, copied and/or
      |  -- disclosed only pursuant to the terms of a valid license
      |  -- agreement with Xilinx, Inc. Xilinx hereby grants you
      |  -- a license to use this text/file solely for design, simulation,
      |  -- implementation and creation of design files limited
      |  -- to Xilinx devices or technologies. Use with non-Xilinx
      |  -- devices or technologies is expressly prohibited and
      |  -- immediately terminates your license unless covered by
      |  -- a separate agreement.
      |  --
      |  -- Xilinx is providing this design, code, or information
      |  -- "as is" solely for use in developing programs and
      |  -- solutions for Xilinx devices. By providing this design,
      |  -- code, or information as one possible implementation of
      |  -- this feature, application or standard, Xilinx is making no
      |  -- representation that this implementation is free from any
      |  -- claims of infringement. You are responsible for
      |  -- obtaining any rights you may require for your implementation.
      |  -- Xilinx expressly disclaims any warranty whatsoever with
      |  -- respect to the adequacy of the implementation, including
      |  -- but not limited to any warranties or representations that this
      |  -- implementation is free from claims of infringement, implied
      |  -- warranties of merchantability or fitness for a particular
      |  -- purpose.
      |  --
      |  -- Xilinx products are not intended for use in life support
      |  -- appliances, devices, or systems. Use in such applications are
      |  -- expressly prohibited.
      |  --
      |  -- This copyright and support notice must be retained as part
      |  -- of this text at all times. (c) Copyright 1995-2005 Xilinx, Inc.
      |  -- All rights reserved.

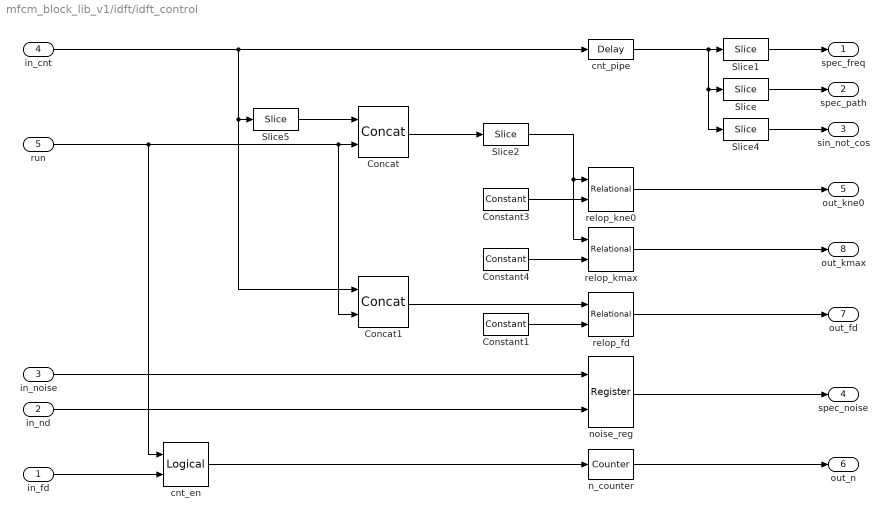
== system mfcm_block_lib_v1/idft/idft_control ==
  in_fd : Inport  Port=1  LatchInput=off
  in_nd : Inport  Port=2  LatchInput=off
  in_noise : Inport  Port=3  LatchInput=off
  in_cnt : Inport  Port=4  LatchInput=off
  run : Inport  Port=5  LatchInput=off
  Concat : xbsIndex_r4/Concat  num_inputs=2  dbl_ovrd=off  block_type=concat
      settings: block_version=VER_STRING_GOES_HERE
  Concat1 : xbsIndex_r4/Concat  num_inputs=2  dbl_ovrd=off  block_type=concat
      settings: block_version=VER_STRING_GOES_HERE
  Constant1 : xbsIndex_r4/Constant  arith_type=Unsigned  const=2*(2^ceil(log2(2*N_OSC*prod(size(SPEC_DATA))))-2*N_OSC*prod(size(SPEC_DATA))+2*N_OSC-2)+1  n_bits=ceil(log2(2*N_OSC*prod(size(SPEC_DATA))))+1  bin_pt=0  explicit_period=off  period=1  equ=P=C  opselect=C  inp2=PCIN>>17  opr=+  inp1=P  carry=CIN  dbl_ovrd=off  block_type=constant
      settings: block_version=VER_STRING_GOES_HERE
  Constant3 : xbsIndex_r4/Constant  arith_type=Unsigned  const=0+1  n_bits=log2(N_OSC)+1  bin_pt=0  explicit_period=off  period=1  equ=P=C  opselect=C  inp2=PCIN>>17  opr=+  inp1=P  carry=CIN  dbl_ovrd=off  block_type=constant
      settings: block_version=VER_STRING_GOES_HERE
  Constant4 : xbsIndex_r4/Constant  arith_type=Unsigned  const=2*(N_OSC-1)+1  n_bits=log2(N_OSC)+1  bin_pt=0  explicit_period=off  period=1  equ=P=C  opselect=C  inp2=PCIN>>17  opr=+  inp1=P  carry=CIN  dbl_ovrd=off  block_type=constant
      settings: block_version=VER_STRING_GOES_HERE
  Slice : xbsIndex_r4/Slice  nbits=ceil(log2(max(prod(size(SPEC_DATA)),2)))  boolean_output=off  mode=Upper Bit Location + Width  bit1=0  base1=MSB of Input  bit0=0  base0=LSB of Input  dbl_ovrd=off  block_type=slice
      settings: infoedit="Extracts a given range of bits from each input sample and presents it at the output.  The output type is ordinarily unsigned with binary point at zero, but can be Boolean when the slice is one bit wide.<P><P>Hardware notes: In hardware this block costs nothing."  block_version=VER_STRING_GOES_HERE
  Slice1 : xbsIndex_r4/Slice  nbits=log2(N_OSC)  boolean_output=off  mode=Lower Bit Location + Width  bit1=0  base1=MSB of Input  bit0=1  base0=LSB of Input  dbl_ovrd=off  block_type=slice
      settings: infoedit="Extracts a given range of bits from each input sample and presents it at the output.  The output type is ordinarily unsigned with binary point at zero, but can be Boolean when the slice is one bit wide.<P><P>Hardware notes: In hardware this block costs nothing."  block_version=VER_STRING_GOES_HERE
  Slice2 : xbsIndex_r4/Slice  nbits=log2(N_OSC)+1  boolean_output=off  mode=Lower Bit Location + Width  bit1=0  base1=MSB of Input  bit0=0  base0=LSB of Input  dbl_ovrd=off  block_type=slice
      settings: infoedit="Extracts a given range of bits from each input sample and presents it at the output.  The output type is ordinarily unsigned with binary point at zero, but can be Boolean when the slice is one bit wide.<P><P>Hardware notes: In hardware this block costs nothing."  block_version=VER_STRING_GOES_HERE
  Slice4 : xbsIndex_r4/Slice  nbits=1  boolean_output=on  mode=Lower Bit Location + Width  bit1=0  base1=MSB of Input  bit0=0  base0=LSB of Input  dbl_ovrd=off  block_type=slice
      settings: infoedit="Extracts a given range of bits from each input sample and presents it at the output.  The output type is ordinarily unsigned with binary point at zero, but can be Boolean when the slice is one bit wide.<P><P>Hardware notes: In hardware this block costs nothing."  block_version=VER_STRING_GOES_HERE
  Slice5 : xbsIndex_r4/Slice  nbits=ceil(log2(prod(size(SPEC_DATA))*N_OSC))  boolean_output=off  mode=Upper Bit Location + Width  bit1=0  base1=MSB of Input  bit0=1  base0=LSB of Input  dbl_ovrd=off  block_type=slice
      settings: infoedit="Extracts a given range of bits from each input sample and presents it at the output.  The output type is ordinarily unsigned with binary point at zero, but can be Boolean when the slice is one bit wide.<P><P>Hardware notes: In hardware this block costs nothing."  block_version=VER_STRING_GOES_HERE
  cnt_en : xbsIndex_r4/Logical  logical_function=AND  inputs=2  en=off  latency=0  precision=Full  arith_type=Unsigned  n_bits=1  bin_pt=0  align_bp=on  dbl_ovrd=off  block_type=logical
      settings: xl_area=[0, 0, 0, 0, 0, 0, 0]  block_version=VER_STRING_GOES_HERE
  cnt_pipe : xbsIndex_r4/Delay  en=off  latency=1  dbl_ovrd=off  reg_retiming=off  block_type=delay
      settings: infoedit="Delay line having  configurable length.<P><P>Hardware notes: A delay line is a chain, each link of which is an SRL16 followed by a flip-flop. If register retiming is enabled, the delay line is a chain of flip-flops."  xl_area=[0, 0, 0, 0, 0, 0, 0]  block_version=VER_STRING_GOES_HERE
  n_counter : xbsIndex_r4/Counter  cnt_type=Free Running  cnt_to=Inf  operation=Up  start_count=0  cnt_by_val=1  arith_type=Unsigned  n_bits=log2(N_IDFT)  bin_pt=0  load_pin=off  rst=off  en=on  dbl_ovrd=off  explicit_period=off  period=1  block_type=counter
      settings: infoedit="Configurable up, down and up/down counter.<P><P>Hardware notes: Free running counters are the least expensive in hardware.  A count limited counter is implemented by combining a counter with a comparator."  block_version=VER_STRING_GOES_HERE
  noise_reg : xbsIndex_r4/Register  init=0  rst=off  en=on  dbl_ovrd=off  block_type=register
      settings: xl_area=[0, 0, 0, 0, 0, 0, 0]  block_version=VER_STRING_GOES_HERE
  relop_fd : xbsIndex_r4/Relational  mode=a=b  en=off  latency=1  dbl_ovrd=off  block_type=relational
      settings: xl_area=[0, 0, 0, 0, 0, 0, 0]  block_version=VER_STRING_GOES_HERE
  relop_kmax : xbsIndex_r4/Relational  mode=a=b  en=off  latency=1  dbl_ovrd=off  block_type=relational
      settings: xl_area=[0, 0, 0, 0, 0, 0, 0]  block_version=VER_STRING_GOES_HERE
  relop_kne0 : xbsIndex_r4/Relational  mode=a!=b  en=off  latency=1  dbl_ovrd=off  block_type=relational
      settings: xl_area=[0, 0, 0, 0, 0, 0, 0]  block_version=VER_STRING_GOES_HERE
  spec_freq : Outport
  spec_path : Outport  Port=2
  sin_not_cos : Outport  Port=3
  spec_noise : Outport  Port=4
  out_kne0 : Outport  Port=5
  out_n : Outport  Port=6
  out_fd : Outport  Port=7
  out_kmax : Outport  Port=8
  wires:
  n_counter/1 -> out_n/1
  in_fd/1 -> cnt_en/2
  cnt_en/1 -> n_counter/1
  Slice4/1 -> sin_not_cos/1
  Concat1/1 -> relop_fd/1
  Slice5/1 -> Concat/1
  Concat/1 -> Slice2/1
  cnt_pipe/1 -> Slice4/1, Slice/1, Slice1/1
  relop_fd/1 -> out_fd/1
  Constant1/1 -> relop_fd/2
  relop_kmax/1 -> out_kmax/1
  Constant4/1 -> relop_kmax/2
  relop_kne0/1 -> out_kne0/1
  Slice2/1 -> relop_kmax/1, relop_kne0/1
  Constant3/1 -> relop_kne0/2
  in_nd/1 -> noise_reg/2
  noise_reg/1 -> spec_noise/1
  in_noise/1 -> noise_reg/1
  Slice/1 -> spec_path/1
  Slice1/1 -> spec_freq/1
  in_cnt/1 -> Concat1/1, Slice5/1, cnt_pipe/1
  run/1 -> cnt_en/1, Concat1/2, Concat/2

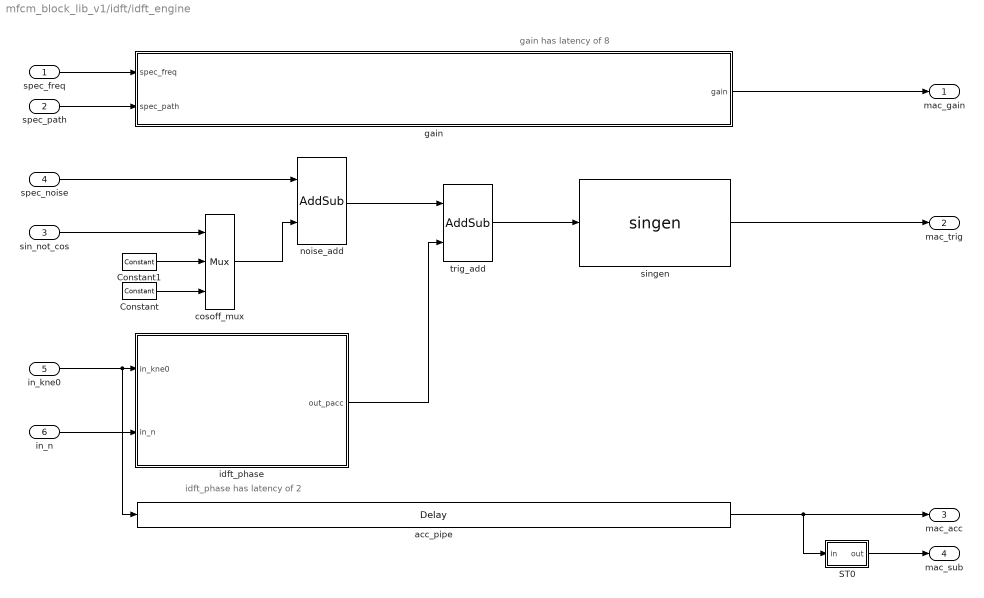
== system mfcm_block_lib_v1/idft/idft_engine ==
  note: idft_phase has latency of 2
  note: gain has latency of 8
  spec_freq : Inport  Port=1  LatchInput=off
  spec_path : Inport  Port=2  LatchInput=off
  sin_not_cos : Inport  Port=3  LatchInput=off
  spec_noise : Inport  Port=4  LatchInput=off
  in_kne0 : Inport  Port=5  LatchInput=off
  in_n : Inport  Port=6  LatchInput=off
  Constant : xbsIndex_r4/Constant  arith_type=Unsigned  const=0  n_bits=log2(N_IDFT)  bin_pt=0  explicit_period=off  period=1  equ=P=C  opselect=C  inp2=PCIN>>17  opr=+  inp1=P  carry=CIN  dbl_ovrd=off  block_type=constant
      settings: block_version=VER_STRING_GOES_HERE
  Constant1 : xbsIndex_r4/Constant  arith_type=Unsigned  const=N_IDFT/4  n_bits=log2(N_IDFT)  bin_pt=0  explicit_period=off  period=1  equ=P=C  opselect=C  inp2=PCIN>>17  opr=+  inp1=P  carry=CIN  dbl_ovrd=off  block_type=constant
      settings: block_version=VER_STRING_GOES_HERE
  ST0 : Subsystem
  acc_pipe : xbsIndex_r4/Delay  en=off  latency=2+1+5  dbl_ovrd=off  reg_retiming=off  block_type=delay
      settings: infoedit="Delay line having  configurable length.<P><P>Hardware notes: A delay line is a chain, each link of which is an SRL16 followed by a flip-flop. If register retiming is enabled, the delay line is a chain of flip-flops."  xl_area=[0, 0, 0, 0, 0, 0, 0]  block_version=VER_STRING_GOES_HERE
  "cosoff_mux " : xbsIndex_r4/Mux  inputs=2  en=off  latency=0  precision=Full  arith_type=Unsigned  n_bits=8  bin_pt=2  quantization=Truncate  overflow=Wrap  dbl_ovrd=off  block_type=mux
      settings: block_version=VER_STRING_GOES_HERE
  gain : Subsystem  mask{ROMS=mfcm_spectrum_roms(SPEC_DATA,N_IDFT)}
      mask prompts: ROMS "Spectrum ROMS"
  idft_phase : Subsystem
  noise_add : xbsIndex_r4/AddSub  mode=Addition  use_carryin=off  use_carryout=off  en=off  latency=2  precision=User Defined  arith_type=Unsigned  n_bits=log2(N_IDFT)  bin_pt=0  quantization=Truncate  overflow=Wrap  dbl_ovrd=off  use_behavioral_HDL=on  pipelined=on  use_rpm=on  block_type=addsub
      settings: xl_area=[0, 0, 0, 0, 0, 0, 0]  block_version=VER_STRING_GOES_HERE
  singen : mfcm_misc_lib_v1/singen  N=N_IDFT  OUT_WIDTH=TRIG_WIDTH  OUT_BINPT=TRIG_WIDTH-1
  trig_add : xbsIndex_r4/AddSub  mode=Addition  use_carryin=off  use_carryout=off  en=off  latency=1  precision=User Defined  arith_type=Unsigned  n_bits=log2(N_IDFT)  bin_pt=0  quantization=Truncate  overflow=Wrap  dbl_ovrd=off  use_behavioral_HDL=on  pipelined=on  use_rpm=on  block_type=addsub
      settings: xl_area=[0, 0, 0, 0, 0, 0, 0]  block_version=VER_STRING_GOES_HERE
  mac_gain : Outport
  mac_trig : Outport  Port=2
  mac_acc : Outport  Port=3
  mac_sub : Outport  Port=4
  wires:
  noise_add/1 -> trig_add/1
  trig_add/1 -> singen/1
  "cosoff_mux "/1 -> noise_add/2
  gain/1(gain) -> mac_gain/1
  Constant/1 -> "cosoff_mux "/3
  Constant1/1 -> "cosoff_mux "/2
  sin_not_cos/1 -> "cosoff_mux "/1
  ST0/1(out) -> mac_sub/1
  acc_pipe/1 -> mac_acc/1, ST0/1(in)
  spec_noise/1 -> noise_add/1
  singen/1 -> mac_trig/1
  spec_path/1 -> gain/2(spec_path)
  spec_freq/1 -> gain/1(spec_freq)
  in_n/1 -> idft_phase/2(in_n)
  in_kne0/1 -> idft_phase/1(in_kne0), acc_pipe/1
  idft_phase/1(out_pacc) -> trig_add/2

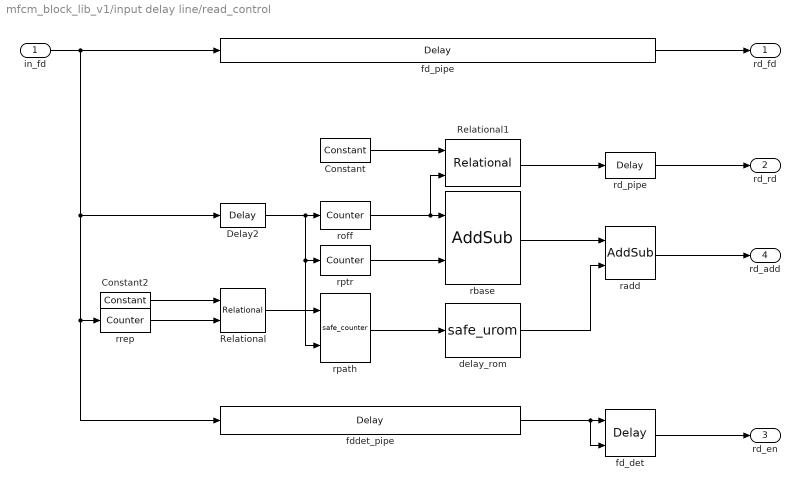
== system mfcm_block_lib_v1/input delay line/read_control ==
  in_fd : Inport  Port=1  LatchInput=off
  Constant : xbsIndex_r4/Constant  arith_type=Unsigned  const=0  n_bits=1  bin_pt=0  explicit_period=off  period=1  equ=P=C  opselect=C  inp2=PCIN>>17  opr=+  inp1=P  carry=CIN  dbl_ovrd=off  block_type=constant
      settings: block_version=VER_STRING_GOES_HERE
  Constant2 : xbsIndex_r4/Constant  arith_type=Unsigned  const=2*MT^2-1  n_bits=ceil(log2(2*MT^2))  bin_pt=0  explicit_period=off  period=1  equ=P=C  opselect=C  inp2=PCIN>>17  opr=+  inp1=P  carry=CIN  dbl_ovrd=off  block_type=constant
      settings: block_version=VER_STRING_GOES_HERE
  Delay2 : xbsIndex_r4/Delay  en=off  latency=1  dbl_ovrd=off  reg_retiming=off  block_type=delay
      settings: infoedit="Delay line having  configurable length.<P><P>Hardware notes: A delay line is a chain, each link of which is an SRL16 followed by a flip-flop. If register retiming is enabled, the delay line is a chain of flip-flops."  xl_area=[0, 0, 0, 0, 0, 0, 0]  block_version=VER_STRING_GOES_HERE
  Relational : xbsIndex_r4/Relational  mode=a=b  en=off  latency=1  dbl_ovrd=off  block_type=relational
      settings: xl_area=[0, 0, 0, 0, 0, 0, 0]  block_version=VER_STRING_GOES_HERE
  Relational1 : xbsIndex_r4/Relational  mode=a=b  en=off  latency=1  dbl_ovrd=off  block_type=relational
      settings: xl_area=[0, 0, 0, 0, 0, 0, 0]  block_version=VER_STRING_GOES_HERE
  delay_rom : mfcm_misc_lib_v1/safe_urom  DEPTH=length(DELAY)  OUT_TYPE=1  OUT_WIDTH=ceil(log2((max(DELAY)+1)*2*MT))  OUT_BINPT=0  INIT=2*MT*DELAY  LATENCY=1  MEM_MAXDEPTH=16
  fd_det : xbsIndex_r4/Delay  en=on  latency=1  dbl_ovrd=off  reg_retiming=off  block_type=delay
      settings: infoedit="Delay line having  configurable length.<P><P>Hardware notes: A delay line is a chain, each link of which is an SRL16 followed by a flip-flop. If register retiming is enabled, the delay line is a chain of flip-flops."  xl_area=[0, 0, 0, 0, 0, 0, 0]  block_version=VER_STRING_GOES_HERE
  fd_pipe : xbsIndex_r4/Delay  en=off  latency=4  dbl_ovrd=off  reg_retiming=off  block_type=delay
      settings: infoedit="Delay line having  configurable length.<P><P>Hardware notes: A delay line is a chain, each link of which is an SRL16 followed by a flip-flop. If register retiming is enabled, the delay line is a chain of flip-flops."  xl_area=[0, 0, 0, 0, 0, 0, 0]  block_version=VER_STRING_GOES_HERE
  fddet_pipe : xbsIndex_r4/Delay  en=off  latency=3  dbl_ovrd=off  reg_retiming=off  block_type=delay
      settings: infoedit="Delay line having  configurable length.<P><P>Hardware notes: A delay line is a chain, each link of which is an SRL16 followed by a flip-flop. If register retiming is enabled, the delay line is a chain of flip-flops."  xl_area=[0, 0, 0, 0, 0, 0, 0]  block_version=VER_STRING_GOES_HERE
  radd : xbsIndex_r4/AddSub  mode=Subtraction  use_carryin=off  use_carryout=off  en=off  latency=1  precision=User Defined  arith_type=Unsigned  n_bits=log2(mfcm_delay_line_depth(DELAY,MT))  bin_pt=0  quantization=Truncate  overflow=Wrap  dbl_ovrd=off  use_behavioral_HDL=on  pipelined=off  use_rpm=on  block_type=addsub
      settings: xl_area=[0, 0, 0, 0, 0, 0, 0]  block_version=VER_STRING_GOES_HERE
  rbase : xbsIndex_r4/AddSub  mode=Addition  use_carryin=off  use_carryout=off  en=off  latency=1  precision=User Defined  arith_type=Unsigned  n_bits=log2(mfcm_delay_line_depth(DELAY,MT))  bin_pt=0  quantization=Truncate  overflow=Wrap  dbl_ovrd=off  use_behavioral_HDL=on  pipelined=off  use_rpm=on  block_type=addsub
      settings: xl_area=[0, 0, 0, 0, 0, 0, 0]  block_version=VER_STRING_GOES_HERE
  rd_pipe : xbsIndex_r4/Delay  en=off  latency=1  dbl_ovrd=off  reg_retiming=off  block_type=delay
      settings: infoedit="Delay line having  configurable length.<P><P>Hardware notes: A delay line is a chain, each link of which is an SRL16 followed by a flip-flop. If register retiming is enabled, the delay line is a chain of flip-flops."  xl_area=[0, 0, 0, 0, 0, 0, 0]  block_version=VER_STRING_GOES_HERE
  roff : xbsIndex_r4/Counter  cnt_type=Count Limited  cnt_to=2*MT-1  operation=Up  start_count=0  cnt_by_val=1  arith_type=Unsigned  n_bits=ceil(log2(2*MT))  bin_pt=0  load_pin=off  rst=on  en=off  dbl_ovrd=off  explicit_period=off  period=1  block_type=counter
      settings: infoedit="Configurable up, down and up/down counter.<P><P>Hardware notes: Free running counters are the least expensive in hardware.  A count limited counter is implemented by combining a counter with a comparator."  xl_area=[0, 0, 0, 0, 0, 0, 0]  block_version=VER_STRING_GOES_HERE
  rpath : mfcm_misc_lib_v1/safe_counter  CNT_MAX=length(DELAY)-1
  rptr : xbsIndex_r4/Counter  cnt_type=Free Running  cnt_to=Inf  operation=Up  start_count=0  cnt_by_val=2*MT  arith_type=Unsigned  n_bits=log2(mfcm_delay_line_depth(DELAY,MT))  bin_pt=0  load_pin=off  rst=off  en=on  dbl_ovrd=off  explicit_period=off  period=1  block_type=counter
      settings: infoedit="Configurable up, down and up/down counter.<P><P>Hardware notes: Free running counters are the least expensive in hardware.  A count limited counter is implemented by combining a counter with a comparator."  xl_area=[0, 0, 0, 0, 0, 0, 0]  block_version=VER_STRING_GOES_HERE
  rrep : xbsIndex_r4/Counter  cnt_type=Count Limited  cnt_to=2*MT^2-1  operation=Up  start_count=0  cnt_by_val=1  arith_type=Unsigned  n_bits=ceil(log2(2*MT^2))  bin_pt=0  load_pin=off  rst=on  en=off  dbl_ovrd=off  explicit_period=off  period=1  block_type=counter
      settings: infoedit="Configurable up, down and up/down counter.<P><P>Hardware notes: Free running counters are the least expensive in hardware.  A count limited counter is implemented by combining a counter with a comparator."  xl_area=[0, 0, 0, 0, 0, 0, 0]  block_version=VER_STRING_GOES_HERE
  rd_fd : Outport
  rd_rd : Outport  Port=2
  rd_en : Outport  Port=3
  rd_add : Outport  Port=4
  wires:
  fddet_pipe/1 -> fd_det/2, fd_det/1
  fd_det/1 -> rd_en/1
  rd_pipe/1 -> rd_rd/1
  rbase/1 -> radd/1
  rptr/1 -> rbase/2
  roff/1 -> Relational1/2, rbase/1
  Delay2/1 -> rpath/2, rptr/1, roff/1
  fd_pipe/1 -> rd_fd/1
  Relational1/1 -> rd_pipe/1
  Constant/1 -> Relational1/1
  Relational/1 -> rpath/1
  Constant2/1 -> Relational/1
  rrep/1 -> Relational/2
  radd/1 -> rd_add/1
  rpath/1 -> delay_rom/1
  in_fd/1 -> fddet_pipe/1, rrep/1, Delay2/1, fd_pipe/1
  delay_rom/1 -> radd/2

== system mfcm_block_lib_v1/input delay line/write_control ==
  in_fd : Inport  Port=1  LatchInput=off
  in_rd : Inport  Port=2  LatchInput=off
  in_reim : Inport  Port=3  LatchInput=off
  Terminator : Terminator
  pulse_extend : mfcm_misc_lib_v1/pulse_extend  WIDTH=2*MT
  reim_pipe : xbsIndex_r4/Delay  en=off  latency=1  dbl_ovrd=off  reg_retiming=off  block_type=delay
      settings: infoedit="Delay line having  configurable length.<P><P>Hardware notes: A delay line is a chain, each link of which is an SRL16 followed by a flip-flop. If register retiming is enabled, the delay line is a chain of flip-flops."  xl_area=[0, 0, 0, 0, 0, 0, 0]  block_version=VER_STRING_GOES_HERE
  wptr : xbsIndex_r4/Counter  cnt_type=Free Running  cnt_to=Inf  operation=Up  start_count=2*MT  cnt_by_val=1  arith_type=Unsigned  n_bits=log2(mfcm_delay_line_depth(DELAY,MT))  bin_pt=0  load_pin=off  rst=off  en=on  dbl_ovrd=off  explicit_period=off  period=1  block_type=counter
      settings: infoedit="Configurable up, down and up/down counter.<P><P>Hardware notes: Free running counters are the least expensive in hardware.  A count limited counter is implemented by combining a counter with a comparator."  xl_area=[0, 0, 0, 0, 0, 0, 0]  block_version=VER_STRING_GOES_HERE
  rd_fd : Outport
  wr_add : Outport  Port=2
  wr_data : Outport  Port=3
  wr_en : Outport  Port=4
  wires:
  in_rd/1 -> Terminator/1
  in_reim/1 -> reim_pipe/1
  pulse_extend/2 -> rd_fd/1
  pulse_extend/1 -> wr_en/1, wptr/1
  in_fd/1 -> pulse_extend/1
  reim_pipe/1 -> wr_data/1
  wptr/1 -> wr_add/1
